simulink model "KDH_simulink"  (R2019b)
settings: Solver=VariableStepAuto  StartTime=0.0  StopTime=10.0  RelTol=1e-3
libraries: dsparch4 x8, dspsnks4 x1, dspsrcs4 x1
settings Model: Creator=jhjh1  LastModifiedBy=jhjh1

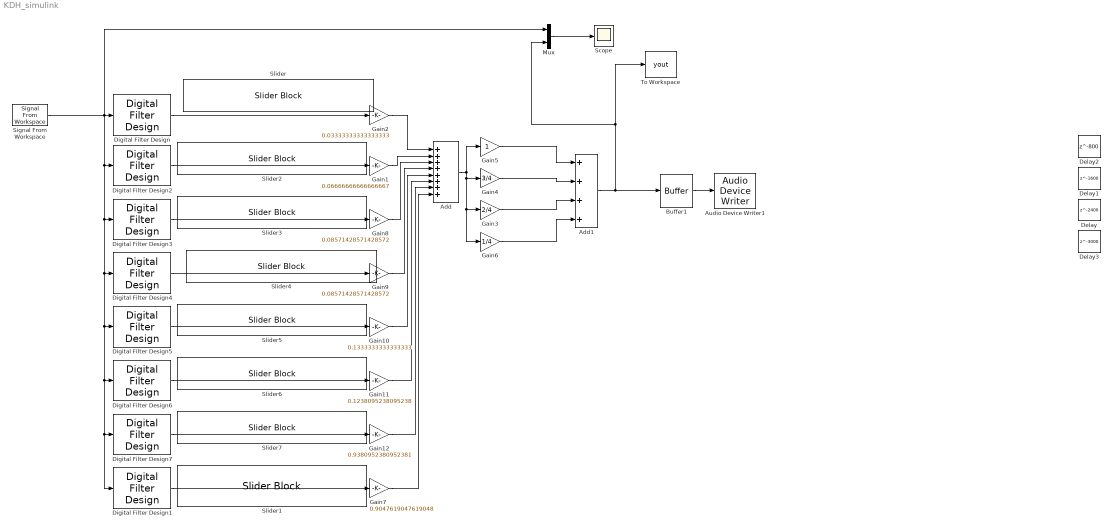
== system KDH_simulink ==
  Add : Sum  Inputs=++++++++
  Add1 : Sum  Inputs=++++
  Audio Device Writer1 : dspsnks4/Audio Device Writer  Driver=DirectSound  Device=Default  InheritSampleRate=on  SampleRate=44100  BitDepth=16-bit integer  BufferSize=4096  NumBuffers=10  DefaultOutputChannelMapping=on  OutputChannelMapping=1:2  OutputNumUnderrunSamples=off  DriverIdx=1  DeviceWarnFlag=''
  Buffer1 : Buffer  N=1024  OutputFrames=off
  Delay : Delay  DelayLength=2400
  Delay1 : Delay  DelayLength=1600
  Delay2 : Delay  DelayLength=800  InitialCondition=0
  Delay3 : Delay  DelayLength=3000
  Digital Filter Design{,1..7} (8 alike) : dsparch4/Digital Filter Design  mwdsp_browser_bugfix_var=off
  Gain1 : Gain  Gain=0.06666666666666667
  Gain10 : Gain  Gain=0.1333333333333333
  Gain11 : Gain  Gain=0.1238095238095238
  Gain12 : Gain  Gain=0.9380952380952381
  Gain2 : Gain  Gain=0.03333333333333333
  Gain3 : Gain  Gain=2/4
  Gain4 : Gain  Gain=3/4
  Gain5 : Gain
  Gain6 : Gain  Gain=1/4
  Gain7 : Gain  Gain=0.9047619047619048
  Gain8 : Gain  Gain=0.08571428571428572
  Gain9 : Gain  Gain=0.08571428571428572
  Mux : Mux  Inputs=2
  Scope : Scope
  Signal From Workspace : dspsrcs4/Signal From Workspace  X=sound_array  Ts=1/48000  nsamps=1  OutputAfterFinalValue=Setting to zero  ignoreOrWarnInputAndFrameLengths=off  OutputFrames=off
  Slider{,1..7} (8 alike) : SliderBlock  ScaleMax=1  TickInterval=0.1
  To Workspace : ToWorkspace  VariableName=yout  SampleTime=-1
      settings: Save2DSignal=2-D array (concatenate along first dimension)
  wires:
  Gain7/1 -> Add/8
  Digital Filter Design/1 -> Gain2/1
  Gain2/1 -> Add/1
  Digital Filter Design1/1 -> Gain7/1
  Buffer1/1 -> Audio Device Writer1/1
  Add/1 -> Gain5/1, Gain6/1, Gain3/1, Gain4/1
  Gain3/1 -> Add1/3
  Gain4/1 -> Add1/2
  Add1/1 -> Buffer1/1, Mux/2, To Workspace/1
  Signal From Workspace/1 -> Digital Filter Design2/1, Digital Filter Design3/1, Digital Filter Design4/1, Digital Filter Design5/1, Digital Filter Design6/1, Digital Filter Design7/1, Digital Filter Design1/1, Mux/1, Digital Filter Design/1
  Gain6/1 -> Add1/4
  Gain5/1 -> Add1/1
  Mux/1 -> Scope/1
  Digital Filter Design2/1 -> Gain1/1
  Digital Filter Design3/1 -> Gain8/1
  Gain8/1 -> Add/3
  Gain1/1 -> Add/2
  Gain9/1 -> Add/4
  Gain10/1 -> Add/5
  Gain11/1 -> Add/6
  Gain12/1 -> Add/7
  Digital Filter Design4/1 -> Gain9/1
  Digital Filter Design5/1 -> Gain10/1
  Digital Filter Design6/1 -> Gain11/1
  Digital Filter Design7/1 -> Gain12/1
